simulink model "exp06"  (R2018a)
settings: Solver=VariableStepAuto  StartTime=0.0  StopTime=10.0  RelTol=1e-3
values from neighbouring files (symbols this model uses):
  B = 0.1    [DCMotor.m]    (also in StateSpace.m = [1;2]; exp05mat.m = [1;2]; exp06matlab.m)
  J = 0.01    [DCMotor.m]    (also in exp06matlab.m)
  K_b = 0.1    [DCMotor.m]    (also in exp06matlab.m)
  K_t = 0.1    [DCMotor.m]    (also in exp06matlab.m)
  L = 0.5    [DCMotor.m]    (also in exp06matlab.m)
  R = 1    [DCMotor.m]    (also in exp06matlab.m)
libraries: simulink x2
settings Model: Creator=SHRUTI  LastModifiedBy=SHRUTI

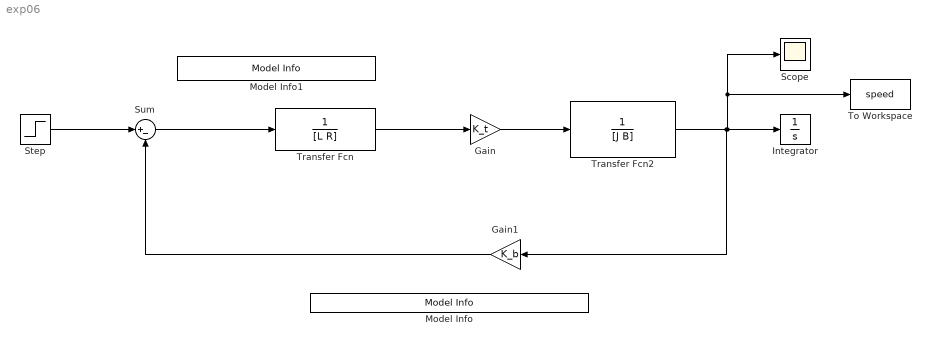
== system exp06 ==
  Gain : Gain  Gain=K_t
  Gain1 : Gain  Gain=K_b
  Integrator : Integrator
  Model Info : simulink/Model-Wide Utilities/Model Info  Frame=on  DisplayStringWithTags=SIMULINK Model to control speed of DC motor.  HorizontalTextAlignment=Center  LeftAlignmentValue=0.5
  Model Info1 : simulink/Model-Wide Utilities/Model Info  Frame=on  DisplayStringWithTags=PRN : 17070123102  HorizontalTextAlignment=Center  LeftAlignmentValue=0.5
  Scope : Scope
  Step : Step  Time=0  SampleTime=0
  Sum : Sum  Inputs=|+-
  To Workspace : ToWorkspace  VariableName=speed  SampleTime=-1
  Transfer Fcn : TransferFcn  Denominator=[L R]
  Transfer Fcn2 : TransferFcn  Denominator=[J B]
  wires:
  Sum/1 -> Transfer Fcn/1
  Transfer Fcn/1 -> Gain/1
  Gain/1 -> Transfer Fcn2/1
  Transfer Fcn2/1 -> Gain1/1, To Workspace/1, Scope/1, Integrator/1
  Gain1/1 -> Sum/2
  Step/1 -> Sum/1
